simulink model "first"  (R2023a)
settings: Solver=FixedStepAuto  StartTime=0.0  StopTime=10  FixedStep=0.001  RelTol=1e-3
settings Model: Creator=evdokiiagalkina  LastModifiedBy=evdokiiagalkina

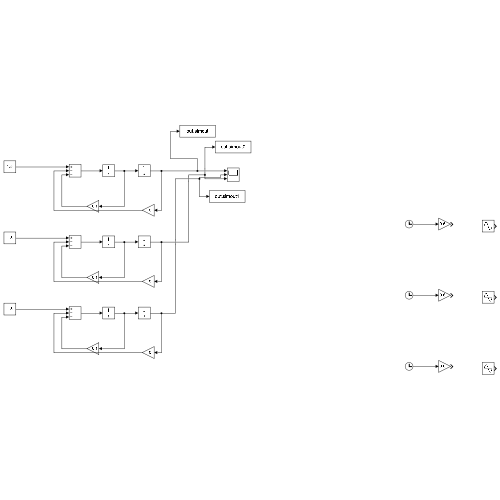
[thumbnail: Simulink's stored preview of the top-level diagram]
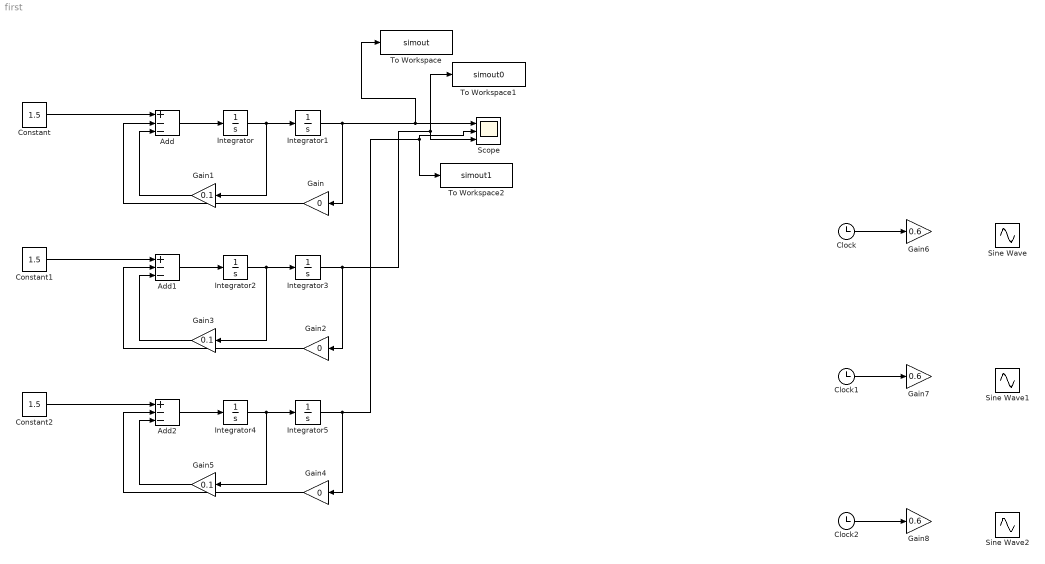
== system first ==
  Add : Sum  Inputs=+--
  Add1 : Sum  Inputs=+--
  Add2 : Sum  Inputs=+--
  Clock : Clock
  Clock1 : Clock
  Clock2 : Clock
  Constant : Constant  Value=1.5  SampleTime=-1
  Constant1 : Constant  Value=1.5  SampleTime=-1
  Constant2 : Constant  Value=1.5  SampleTime=-1
  Gain : Gain  Gain=0
  Gain1 : Gain  Gain=0.1
  Gain2 : Gain  Gain=0
  Gain3 : Gain  Gain=0.1
  Gain4 : Gain  Gain=0
  Gain5 : Gain  Gain=0.1
  Gain6 : Gain  Gain=0.6
  Gain7 : Gain  Gain=0.6
  Gain8 : Gain  Gain=0.6
  Integrator{,2..4} (4 alike) : Integrator
  Integrator1 : Integrator  InitialCondition=-1
  Integrator5 : Integrator  InitialCondition=1
  Scope : Scope  NumInputPorts=3
  Sine Wave : Sin  Amplitude=6  SampleTime=0
  Sine Wave1 : Sin  Amplitude=6  SampleTime=0
  Sine Wave2 : Sin  Amplitude=6  SampleTime=0
  To Workspace : ToWorkspace  VariableName=simout  SaveFormat=Timeseries  SampleTime=-1
  To Workspace1 : ToWorkspace  VariableName=simout0  SaveFormat=Timeseries  SampleTime=-1
  To Workspace2 : ToWorkspace  VariableName=simout1  SaveFormat=Timeseries  SampleTime=-1
  wires:
  Integrator/1 -> Gain1/1, Integrator1/1
  Constant/1 -> Add/1
  Add/1 -> Integrator/1
  Integrator1/1 -> Gain/1, Scope/1, To Workspace/1
  Gain1/1 -> Add/3
  Gain/1 -> Add/2
  Integrator2/1 -> Gain3/1, Integrator3/1
  Gain2/1 -> Add1/2
  Gain3/1 -> Add1/3
  Integrator3/1 -> Scope/3, To Workspace1/1, Gain2/1
  Constant1/1 -> Add1/1
  Add1/1 -> Integrator2/1
  Integrator4/1 -> Gain5/1, Integrator5/1
  Gain4/1 -> Add2/2
  Gain5/1 -> Add2/3
  Integrator5/1 -> Scope/2, To Workspace2/1, Gain4/1
  Constant2/1 -> Add2/1
  Add2/1 -> Integrator4/1
  Clock2/1 -> Gain8/1
  Clock1/1 -> Gain7/1
  Clock/1 -> Gain6/1
